simulink model "TEST_IPM_2_0"  (R2019b)
settings: configuration reference "Configuration" (kept outside this file)
PreLoadFcn:
  | RTWConfigurationCB('preloadfcn', bdroot);
values from neighbouring files (symbols this model uses):
  MParamFbase = 200.0    [TEST_IPM_LIB.sldd]
  MParamIbase = 360.0    [TEST_IPM_LIB.sldd]
  MParamLd = 0.002    [TEST_IPM_LIB.sldd]
  MParamLq = 0.002    [TEST_IPM_LIB.sldd]
  MParamRs = 1.15    [TEST_IPM_LIB.sldd]
  PWM_TPBRD_HALF = 5000.0    [TEST_IPM_LIB.sldd]
  Ts_10kHz = 0.0001    [TEST_IPM_LIB.sldd]
  Ts_1kHz = 0.001    [TEST_IPM_LIB.sldd]
undefined symbols (not defined in the file or in its folder): Down, GPTRIP1SEL, GPTRIP2SEL, TZ1, TZ2, Up
libraries: c280xlib x66, c2837xDlib x18, c2802xlib x10, powerlib_meascontrol x9, dsparch4 x4, c2000lib x1, c2806xlib x1, idelinklib_common x1
(part 5 of 6)

== system TEST_IPM_2_0/INT/Read Rotor Position/SpeedCal1 ==
  In1 : Inport
  function : TriggerPort  TriggerType=function-call  VariantControl=Variant
  "First Order Filter " : Subsystem
  MATLAB Function1 : MATLAB Function  TreatAsAtomicUnit=on
  Unit Delay : UnitDelay  SampleTime=-1  HasFrameUpgradeWarning=on
  Out1 : Outport
  wires:
  In1/1 -> Unit Delay/1, MATLAB Function1/1(theta)
  Unit Delay/1 -> MATLAB Function1/2(theta_old)
  MATLAB Function1/1(speed) -> "First Order Filter "/1(input)
  "First Order Filter "/1("output ") -> Out1/1

== system TEST_IPM_2_0/INT/ePWM/If Action Subsystem ==
  Action Port : ActionPort  ActionPortLabel=if(u1 == 1)
  Constant : Constant  Value=0  OutDataTypeStr=single  SampleTime=-1
  Data Store Write : DataStoreWrite  DataStoreName=N_Integral
  Data Store Write1 : DataStoreWrite  DataStoreName=Iq_Integral
  Data Store Write2 : DataStoreWrite  DataStoreName=Id_Integral
  Data Store Write3 : DataStoreWrite  DataStoreName=PLL_Integral
  Data Store Write4 : DataStoreWrite  DataStoreName=Theta_Integral
  wires:
  Constant/1 -> Data Store Write3/1, Data Store Write4/1, Data Store Write1/1, Data Store Write2/1, Data Store Write/1

== system TEST_IPM_2_0/INT/Motor Control/Current_PI/PID_Id  ==
  Ref : Inport
  Fbk : Inport  Port=2
  Data Store Read : DataStoreRead  DataStoreName=Id_Kp
  Data Store Read1 : DataStoreRead  DataStoreName=Id_Integral
  Data Store Read3 : DataStoreRead  DataStoreName=UDCPROTECT
  Data Store Write : DataStoreWrite  DataStoreName=Id_Integral
  MATLAB Function1 : MATLAB Function  TreatAsAtomicUnit=on
  Product : Product  OutDataTypeStr=Inherit: Same as first input
  Subsystem : Subsystem
  Sum1 : Sum  OutDataTypeStr=single
  Sum2 : Sum  Inputs=+-  OutDataTypeStr=Inherit: Inherit via back propagation
  Out : Outport
  wires:
  Data Store Read1/1 -> Subsystem/1(OLD_UI_REG3)
  Fbk/1 -> Sum2/2
  Ref/1 -> Sum2/1
  Product/1 -> Sum1/1
  Data Store Read/1 -> Product/2
  Sum2/1 -> Subsystem/2(up_reg3), Product/1
  Sum1/1 -> Out/1
  Data Store Read3/1 -> MATLAB Function1/1(Udc)
  Subsystem/1(UI_REG1) -> MATLAB Function1/2(Input), Sum1/2
  MATLAB Function1/1(Output) -> Data Store Write/1

== system TEST_IPM_2_0/INT/Motor Control/Current_PI/PID_Iq ==
  Ref : Inport
  Fbk : Inport  Port=2
  Data Store Read : DataStoreRead  DataStoreName=Iq_Kp
  Data Store Read1 : DataStoreRead  DataStoreName=Iq_Integral
  Data Store Read2 : DataStoreRead  DataStoreName=UDCPROTECT
  Data Store Read3 : DataStoreRead  DataStoreName=UDCPROTECT
  Data Store Write : DataStoreWrite  DataStoreName=Iq_Integral
  MATLAB Function : MATLAB Function  TreatAsAtomicUnit=on
  MATLAB Function1 : MATLAB Function  TreatAsAtomicUnit=on
  Product : Product  OutDataTypeStr=Inherit: Same as first input
  Subsystem : Subsystem
  Sum1 : Sum  OutDataTypeStr=single
  Sum2 : Sum  Inputs=+-  OutDataTypeStr=Inherit: Inherit via back propagation
  Out : Outport
  wires:
  MATLAB Function1/1(Output) -> Data Store Write/1
  Subsystem/1(UI_REG1) -> Sum1/2, MATLAB Function1/2(Input)
  Data Store Read3/1 -> MATLAB Function1/1(Udc)
  MATLAB Function/1(Output) -> Out/1
  Data Store Read2/1 -> MATLAB Function/1(Udc)
  Sum1/1 -> MATLAB Function/2(Input)
  Sum2/1 -> Product/1, Subsystem/2(up_reg3)
  Data Store Read/1 -> Product/2
  Product/1 -> Sum1/1
  Ref/1 -> Sum2/1
  Fbk/1 -> Sum2/2
  Data Store Read1/1 -> Subsystem/1(OLD_UI_REG3)

== system TEST_IPM_2_0/INT/Motor Control/Current_PI/RealVoltageCompesation  ==
  Udq : Inport
  Iuvw : Inport  Port=2
  Add : Sum  Inputs=+-
  Add1 : Sum  Inputs=+-
  Add2 : Sum  AccumDataTypeStr=single  OutDataTypeStr=single
  Clark Transformation : Subsystem
  Data Store Read : DataStoreRead  DataStoreName=K
  Data Store Read1 : DataStoreRead  DataStoreName=Udelta
  Data Store Read2 : DataStoreRead  DataStoreName=ControlAng
  Data Store Read3 : DataStoreRead  DataStoreName=N_REF
  Data Store Read4 : DataStoreRead  DataStoreName=DEKF_Udelay
  Data Store Read5 : DataStoreRead  DataStoreName=Alpha_Current
  Data Store Read6 : DataStoreRead  DataStoreName=Beta_Current
  Delay : Delay
  Demux : Demux  Outputs=3
  Demux1 : Demux  Outputs=2
  Gain : Gain  Gain=5/60*2*pi*1e-4
  MATLAB Function : MATLAB Function  TreatAsAtomicUnit=on
  MATLAB Function1 : MATLAB Function  TreatAsAtomicUnit=on
  MATLAB Function2 : MATLAB Function  TreatAsAtomicUnit=on
  Park Transformation : Subsystem
  Park Transformation1 : Subsystem
  Product : Product
  Sqrt : Sqrt  OutputSignalType=real  OutDataTypeStr=single  IntermediateResultsDataTypeStr=single  SaturateOnIntegerOverflow=on
  Square : Math  Operator=square  SignedPower=off  OutputSignalType=real  OutDataTypeStr=single  SaturateOnIntegerOverflow=on
  Square1 : Math  Operator=square  SignedPower=off  OutputSignalType=real  OutDataTypeStr=single  SaturateOnIntegerOverflow=on
  Subsystem : Subsystem
  UdComP : Outport
  UqComP : Outport  Port=2
  UsComP : Outport  Port=3
  wires:
  Udq/1 -> Delay/1
  Demux/1 -> MATLAB Function/1(I)
  Demux/2 -> MATLAB Function1/1(I)
  Demux/3 -> MATLAB Function2/1(I)
  Data Store Read/1 -> MATLAB Function2/2(K), MATLAB Function1/2(K), MATLAB Function/2(K)
  Data Store Read1/1 -> MATLAB Function/3(Udead), MATLAB Function1/3(Udead), MATLAB Function2/3(Udead)
  MATLAB Function/1(Uerror) -> Clark Transformation/1(U)
  MATLAB Function1/1(Uerror) -> Clark Transformation/2(V)
  MATLAB Function2/1(Uerror) -> Clark Transformation/3(W)
  Clark Transformation/2(Beta) -> Park Transformation/2(Beta)
  Delay/1 -> Demux1/1
  Park Transformation/1(D) -> Add/2
  Park Transformation/2(Q) -> Add1/2
  Data Store Read3/1 -> Gain/1
  Demux1/1 -> Park Transformation1/1(Alpha)
  Demux1/2 -> Park Transformation1/2(Beta)
  Sqrt/1 -> UsComP/1
  Square1/1 -> Add2/2
  Add/1 -> Square/1, Subsystem/1(Ud), UdComP/1
  Square/1 -> Add2/1
  Add1/1 -> Subsystem/2(Uq), Square1/1, UqComP/1
  Add2/1 -> Sqrt/1
  Park Transformation1/1(D) -> Add/1
  Park Transformation1/2(Q) -> Add1/1
  Iuvw/1 -> Demux/1
  Data Store Read2/1 -> Subsystem/5(Theta), Park Transformation/3(theta)
  Product/1 -> Park Transformation1/3(theta)
  Gain/1 -> Product/1
  Data Store Read4/1 -> Product/2
  Clark Transformation/1(Alpha) -> Park Transformation/1(Alpha)
  Data Store Read5/1 -> Subsystem/3(Ial)
  Data Store Read6/1 -> Subsystem/4(Ibe)

== system TEST_IPM_2_0/INT/Motor Control/IF/Subsystem1 ==
  TargetValue : Inport
  Step : Inport  Port=2
  MATLAB Function : MATLAB Function  TreatAsAtomicUnit=on
  Unit Delay : UnitDelay  SampleTime=-1  HasFrameUpgradeWarning=on
  RampOutput : Outport
  wires:
  TargetValue/1 -> MATLAB Function/1(Target)
  MATLAB Function/1(Output) -> RampOutput/1, Unit Delay/1
  Step/1 -> MATLAB Function/2(Step)
  Unit Delay/1 -> MATLAB Function/3(LastOutput)

== system TEST_IPM_2_0/INT/Motor Control/IF/Subsystem2 ==
  FRQ : Inport
  MATLAB Function : MATLAB Function  TreatAsAtomicUnit=on
  Unit Delay : UnitDelay  SampleTime=-1  HasFrameUpgradeWarning=on
  Ang : Outport
  wires:
  MATLAB Function/1(Ang) -> Ang/1, Unit Delay/1
  Unit Delay/1 -> MATLAB Function/2(LastAng)
  FRQ/1 -> MATLAB Function/1(FRQ)

== system TEST_IPM_2_0/INT/Motor Control/SVPWM/Inverse Park Transformation ==
  D : Inport
  Q : Inport  Port=2
  theta : Inport  Port=3
  Product{,1..3} (4 alike) : Product  OutDataTypeStr=Inherit: Same as first input
  Sin : Trigonometry  OutputSignalType=real
  Sin1 : Trigonometry  Operator=cos  OutputSignalType=real
  Sum1 : Sum  Inputs=|++  OutDataTypeStr=Inherit: Same as first input
  Sum2 : Sum  Inputs=|+-  OutDataTypeStr=Inherit: Same as first input
  Alpha : Outport
  Beta : Outport  Port=2
  wires:
  Sin1/1 -> Product2/2, Product/2
  Sin/1 -> Product3/2, Product1/2
  Product3/1 -> Sum1/2
  Sum1/1 -> Beta/1
  D/1 -> Product3/1, Product/1
  Product2/1 -> Sum1/1
  Sum2/1 -> Alpha/1
  Product/1 -> Sum2/1
  Product1/1 -> Sum2/2
  Q/1 -> Product2/1, Product1/1
  theta/1 -> Sin/1, Sin1/1

== system TEST_IPM_2_0/INT/Motor Control/SpeedMode/Function-Call Subsystem ==
  function : TriggerPort  TriggerType=function-call  VariantControl=Variant
  Constant : Constant  Value=0  OutDataTypeStr=single  SampleTime=-1
  Constant1 : Constant  Value=0  OutDataTypeStr=single  SampleTime=-1
  Data Store Read1 : DataStoreRead  DataStoreName=N_FBK
  Data Store Read2 : DataStoreRead  DataStoreName=STOP
  Data Store Read3 : DataStoreRead  DataStoreName=N_REF
  Data Store Read5 : DataStoreRead  DataStoreName=FLAG_MTPA
  Data Store Write1 : DataStoreWrite  DataStoreName=Iq_REF
  Demux : Demux  Outputs=2
  If Action Subsystem : Subsystem  TreatAsAtomicUnit=on
  MATLAB Function : MATLAB Function  TreatAsAtomicUnit=on
  Mux : Mux  Inputs=2
  Mux1 : Mux  Inputs=2
  "PID_n " : Subsystem
  Switch : Switch  Criteria=u2 ~= 0
  wires:
  Constant/1 -> Mux1/1
  Constant1/1 -> Mux1/2
  Switch/1 -> Demux/1
  Data Store Read1/1 -> Mux/2
  Demux/2 -> "PID_n "/2(Fbk)
  Demux/1 -> "PID_n "/1(Ref)
  Mux1/1 -> Switch/1
  Data Store Read2/1 -> Switch/2
  Data Store Read3/1 -> Mux/1
  Mux/1 -> Switch/3
  "PID_n "/1(Out) -> Data Store Write1/1
  Data Store Read5/1 -> MATLAB Function/1(FLAG)
  MATLAB Function/1(FcnCal()) -> If Action Subsystem/Trigger

== system TEST_IPM_2_0/INT/Motor Control/TorqueMode/Function-Call Subsystem ==
  function : TriggerPort  TriggerType=function-call  VariantControl=Variant
  Constant : Constant  Value=0  OutDataTypeStr=single  SampleTime=-1
  Constant1 : Constant  Value=0  OutDataTypeStr=single  SampleTime=-1
  Constant2 : Constant  Value=0  OutDataTypeStr=single  SampleTime=-1
  Data Store Write : DataStoreWrite  DataStoreName=N_Integral
  Data Store Write1 : DataStoreWrite  DataStoreName=Iq_Integral
  Data Store Write2 : DataStoreWrite  DataStoreName=Id_Integral
  wires:
  Constant1/1 -> Data Store Write2/1
  Constant2/1 -> Data Store Write1/1
  Constant/1 -> Data Store Write/1

== system TEST_IPM_2_0/INT/Motor Control/VF/Subsystem1 ==
  TargetValue : Inport
  Step : Inport  Port=2
  MATLAB Function : MATLAB Function  TreatAsAtomicUnit=on
  Unit Delay : UnitDelay  SampleTime=-1  HasFrameUpgradeWarning=on
  RampOutput : Outport
  wires:
  TargetValue/1 -> MATLAB Function/1(Target)
  MATLAB Function/1(Output) -> RampOutput/1, Unit Delay/1
  Step/1 -> MATLAB Function/2(Step)
  Unit Delay/1 -> MATLAB Function/3(LastOutput)

== system TEST_IPM_2_0/INT/Motor Control/VF/Subsystem2 ==
  FRQ : Inport
  MATLAB Function : MATLAB Function  TreatAsAtomicUnit=on
  Unit Delay : UnitDelay  SampleTime=-1  HasFrameUpgradeWarning=on
  Ang : Outport
  wires:
  MATLAB Function/1(Ang) -> Ang/1, Unit Delay/1
  Unit Delay/1 -> MATLAB Function/2(LastAng)
  FRQ/1 -> MATLAB Function/1(FRQ)

== system TEST_IPM_2_0/INT/Read Rotor Position/SpeedCal/First Order Filter  ==
  input : Inport
  Add : Sum  Inputs=+-
  Add3 : Sum  AccumDataTypeStr=single
  Constant : Constant  OutDataTypeStr=single  SampleTime=-1
  Data Store Read1 : DataStoreRead  DataStoreName=N_Filter
  Data Store Read2 : DataStoreRead  DataStoreName=N_Filter
  Gain : Gain  Gain=2*pi*Ts_1kHz
  Gain1 : Gain  Gain=2*pi*Ts_1kHz
  Product : Product
  Product1 : Product
  Unit Delay3 : UnitDelay  SampleTime=-1  HasFrameUpgradeWarning=on
  "output " : Outport
  wires:
  input/1 -> Product/1
  Product/1 -> Add3/1
  Product1/1 -> Unit Delay3/1
  Add3/1 -> Product1/1, "output "/1
  Unit Delay3/1 -> Add3/2
  Data Store Read2/1 -> Gain/1
  Gain/1 -> Product/2
  Data Store Read1/1 -> Gain1/1
  Add/1 -> Product1/2
  Gain1/1 -> Add/2
  Constant/1 -> Add/1

== system TEST_IPM_2_0/INT/Read Rotor Position/SpeedCal1/First Order Filter  ==
  input : Inport
  Add : Sum  Inputs=+-
  Add3 : Sum  AccumDataTypeStr=single
  Constant : Constant  OutDataTypeStr=single  SampleTime=-1
  Data Store Read1 : DataStoreRead  DataStoreName=N_Filter
  Data Store Read2 : DataStoreRead  DataStoreName=N_Filter
  Gain : Gain  Gain=2*pi*Ts_1kHz
  Gain1 : Gain  Gain=2*pi*Ts_1kHz
  Product : Product
  Product1 : Product
  Unit Delay3 : UnitDelay  SampleTime=-1  HasFrameUpgradeWarning=on
  "output " : Outport
  wires:
  input/1 -> Product/1
  Product/1 -> Add3/1
  Product1/1 -> Unit Delay3/1
  Add3/1 -> Product1/1, "output "/1
  Unit Delay3/1 -> Add3/2
  Data Store Read2/1 -> Gain/1
  Gain/1 -> Product/2
  Data Store Read1/1 -> Gain1/1
  Add/1 -> Product1/2
  Gain1/1 -> Add/2
  Constant/1 -> Add/1

== system TEST_IPM_2_0/INT/Motor Control/Current_PI/PID_Id /Subsystem ==
  OLD_UI_REG3 : Inport
  up_reg3 : Inport  Port=2
  Data Store Read2 : DataStoreRead  DataStoreName=Id_Ki
  Gain : Gain  Gain=Ts_10kHz
  Product1 : Product  OutDataTypeStr=Inherit: Same as first input
  Sum3 : Sum
  UI_REG1 : Outport
  wires:
  Sum3/1 -> UI_REG1/1
  up_reg3/1 -> Product1/2
  Product1/1 -> Sum3/2
  OLD_UI_REG3/1 -> Sum3/1
  Gain/1 -> Product1/1
  Data Store Read2/1 -> Gain/1

== system TEST_IPM_2_0/INT/Motor Control/Current_PI/PID_Iq/Subsystem ==
  OLD_UI_REG3 : Inport
  up_reg3 : Inport  Port=2
  Data Store Read2 : DataStoreRead  DataStoreName=Iq_Ki
  Gain : Gain  Gain=Ts_10kHz
  Product1 : Product  OutDataTypeStr=Inherit: Same as first input
  Sum3 : Sum
  UI_REG1 : Outport
  wires:
  Data Store Read2/1 -> Gain/1
  Gain/1 -> Product1/1
  OLD_UI_REG3/1 -> Sum3/1
  Product1/1 -> Sum3/2
  up_reg3/1 -> Product1/2
  Sum3/1 -> UI_REG1/1

== system TEST_IPM_2_0/INT/Motor Control/Current_PI/RealVoltageCompesation /Clark Transformation ==
  U : Inport
  V : Inport  Port=2
  W : Inport  Port=3
  Add : Sum  Inputs=+--
  Add1 : Sum  Inputs=+-
  Gain : Gain  Gain=0.5
  Gain1 : Gain  Gain=0.5
  Gain2 : Gain  Gain=2/3
  Gain3 : Gain  Gain=2/3*0.86602540
  Alpha : Outport
  Beta : Outport  Port=2
  wires:
  V/1 -> Add1/1, Gain/1
  Gain/1 -> Add/2
  W/1 -> Add1/2, Gain1/1
  Gain1/1 -> Add/3
  U/1 -> Add/1
  Add/1 -> Gain2/1
  Gain2/1 -> Alpha/1
  Add1/1 -> Gain3/1
  Gain3/1 -> Beta/1

== system TEST_IPM_2_0/INT/Motor Control/Current_PI/RealVoltageCompesation /Park Transformation ==
  Alpha : Inport
  Beta : Inport  Port=2
  theta : Inport  Port=3
  Add : Sum
  Add1 : Sum  Inputs=+-
  Product{,1..3} (4 alike) : Product
  Sin : Trigonometry  OutputSignalType=real
  Sin1 : Trigonometry  Operator=cos  OutputSignalType=real
  D : Outport
  Q : Outport  Port=2
  wires:
  Product/1 -> Add/1
  Sin/1 -> Product3/2, Product1/2
  Product1/1 -> Add/2
  Add1/1 -> Q/1
  Sin1/1 -> Product2/2, Product/2
  Product2/1 -> Add1/1
  Alpha/1 -> Product3/1, Product/1
  Beta/1 -> Product2/1, Product1/1
  Product3/1 -> Add1/2
  Add/1 -> D/1
  theta/1 -> Sin/1, Sin1/1

== system TEST_IPM_2_0/INT/Motor Control/Current_PI/RealVoltageCompesation /Park Transformation1 ==
  Alpha : Inport
  Beta : Inport  Port=2
  theta : Inport  Port=3
  Add : Sum
  Add1 : Sum  Inputs=+-
  Product{,1..3} (4 alike) : Product
  Sin : Trigonometry  OutputSignalType=real
  Sin1 : Trigonometry  Operator=cos  OutputSignalType=real
  D : Outport
  Q : Outport  Port=2
  wires:
  theta/1 -> Sin1/1, Sin/1
  Add/1 -> D/1
  Product3/1 -> Add1/2
  Beta/1 -> Product1/1, Product2/1
  Alpha/1 -> Product/1, Product3/1
  Product2/1 -> Add1/1
  Sin1/1 -> Product/2, Product2/2
  Add1/1 -> Q/1
  Product1/1 -> Add/2
  Sin/1 -> Product1/2, Product3/2
  Product/1 -> Add/1

== system TEST_IPM_2_0/INT/Motor Control/Current_PI/RealVoltageCompesation /Subsystem ==
  Ud : Inport
  Uq : Inport  Port=2
  Ial : Inport  Port=3
  Ibe : Inport  Port=4
  Theta : Inport  Port=5
  Data Store Read : DataStoreRead  DataStoreName=SMO_EalEstOut
  Data Store Read1 : DataStoreRead  DataStoreName=SMO_EbeEstOut
  Data Store Read2 : DataStoreRead  DataStoreName=ResloverAng
  Data Store Write : DataStoreWrite  DataStoreName=SMO_Ual
  Data Store Write1 : DataStoreWrite  DataStoreName=SMO_Ube
  Data Store Write11 : DataStoreWrite  DataStoreName=SMO_Theta
  Data Store Write2 : DataStoreWrite  DataStoreName=SMO_Ial
  Data Store Write3 : DataStoreWrite  DataStoreName=SMO_Ibe
  Data Store Write4 : DataStoreWrite  DataStoreName=SMO_Error
  Data Store Write5 : DataStoreWrite  DataStoreName=SMO_EamEst
  Inverse Park Transformation : Subsystem
  MATLAB Function3 : MATLAB Function  TreatAsAtomicUnit=on
      settings: RTWSystemCode=Inline
  wires:
  Inverse Park Transformation/2(Beta) -> Data Store Write1/1
  MATLAB Function3/1(Theta) -> Data Store Write11/1
  Uq/1 -> Inverse Park Transformation/2(Q)
  Ibe/1 -> Data Store Write3/1
  Inverse Park Transformation/1(Alpha) -> Data Store Write/1
  Ial/1 -> Data Store Write2/1
  Theta/1 -> Inverse Park Transformation/3(theta)
  Ud/1 -> Inverse Park Transformation/1(D)
  Data Store Read2/1 -> MATLAB Function3/3(ControlAng)
  MATLAB Function3/2(Error) -> Data Store Write4/1
  MATLAB Function3/3(Eam) -> Data Store Write5/1
  Data Store Read/1 -> MATLAB Function3/1(Eal)
  Data Store Read1/1 -> MATLAB Function3/2(Ebe)

== system TEST_IPM_2_0/INT/Motor Control/SpeedMode/Function-Call Subsystem/If Action Subsystem ==
  function : TriggerPort  TriggerType=function-call  VariantControl=Variant
  Abs : Abs
  Data Store Read : DataStoreRead  DataStoreName=MTPA_Gamma
  Data Store Read3 : DataStoreRead  DataStoreName=Iq_REF
  Data Store Write1 : DataStoreWrite  DataStoreName=Iq_REF
  Data Store Write2 : DataStoreWrite  DataStoreName=Id_REF
  Gain1 : Gain  Gain=-1  OutDataTypeStr=single
  Product : Product  OutDataTypeStr=single
  Product1 : Product  OutDataTypeStr=single
  Saturation : Saturate  UpperLimit=pi/2  LowerLimit=0
  cos : Trigonometry  Operator=cos  OutputSignalType=real
  sin : Trigonometry  OutputSignalType=real
  wires:
  sin/1 -> Product1/1
  Abs/1 -> Gain1/1
  cos/1 -> Product/2
  Saturation/1 -> sin/1, cos/1
  Product/1 -> Data Store Write1/1
  Gain1/1 -> Product1/2
  Data Store Read3/1 -> Abs/1, Product/1
  Product1/1 -> Data Store Write2/1
  Data Store Read/1 -> Saturation/1

== system TEST_IPM_2_0/INT/Motor Control/SpeedMode/Function-Call Subsystem/PID_n  ==
  Ref : Inport
  Fbk : Inport  Port=2
  Constant : Constant  Value=MParamIbase  OutDataTypeStr=single  SampleTime=-1
  Data Store Read : DataStoreRead  DataStoreName=N_Kp
  Data Store Read1 : DataStoreRead  DataStoreName=N_Integral
  Data Store Write : DataStoreWrite  DataStoreName=N_Integral
  MATLAB Function : MATLAB Function  TreatAsAtomicUnit=on
  Product : Product  OutDataTypeStr=Inherit: Same as first input
  Subsystem : Subsystem
  Sum1 : Sum  OutDataTypeStr=single
  Sum2 : Sum  Inputs=+-  OutDataTypeStr=Inherit: Inherit via back propagation
  Out : Outport
  wires:
  Data Store Read1/1 -> Subsystem/1(OLD_UI_REG3)
  Fbk/1 -> Sum2/2
  Ref/1 -> Sum2/1
  Product/1 -> Sum1/1
  Data Store Read/1 -> Product/2
  Subsystem/1(UI_REG1) -> Data Store Write/1, Sum1/2
  Sum2/1 -> Subsystem/2(up_reg3), Product/1
  MATLAB Function/1(Output) -> Out/1
  Sum1/1 -> MATLAB Function/2(Input)
  Constant/1 -> MATLAB Function/1(Limit)

== system TEST_IPM_2_0/INT/Motor Control/Current_PI/RealVoltageCompesation /Subsystem/Inverse Park Transformation ==
  D : Inport
  Q : Inport  Port=2
  theta : Inport  Port=3
  Product{,1..3} (4 alike) : Product  OutDataTypeStr=Inherit: Same as first input
  Sin : Trigonometry  OutputSignalType=real
  Sin1 : Trigonometry  Operator=cos  OutputSignalType=real
  Sum1 : Sum  Inputs=|++  OutDataTypeStr=Inherit: Same as first input
  Sum2 : Sum  Inputs=|+-  OutDataTypeStr=Inherit: Same as first input
  Alpha : Outport
  Beta : Outport  Port=2
  wires:
  Sin1/1 -> Product2/2, Product/2
  Sin/1 -> Product3/2, Product1/2
  Product3/1 -> Sum1/2
  Sum1/1 -> Beta/1
  D/1 -> Product3/1, Product/1
  Product2/1 -> Sum1/1
  Sum2/1 -> Alpha/1
  Product/1 -> Sum2/1
  Product1/1 -> Sum2/2
  Q/1 -> Product2/1, Product1/1
  theta/1 -> Sin/1, Sin1/1

== system TEST_IPM_2_0/INT/Motor Control/SpeedMode/Function-Call Subsystem/PID_n /Subsystem ==
  OLD_UI_REG3 : Inport
  up_reg3 : Inport  Port=2
  Data Store Read2 : DataStoreRead  DataStoreName=N_Ki
  Gain : Gain  Gain=Ts_1kHz
  Product1 : Product  OutDataTypeStr=Inherit: Same as first input
  Sum3 : Sum  OutDataTypeStr=single
  UI_REG1 : Outport
  wires:
  Sum3/1 -> UI_REG1/1
  up_reg3/1 -> Product1/2
  Product1/1 -> Sum3/2
  OLD_UI_REG3/1 -> Sum3/1
  Gain/1 -> Product1/1
  Data Store Read2/1 -> Gain/1

== stateflow chart TEST_IPM_2_0/INT/AD2S1210 Init/AD2S1210 ==
  settings: updateMethod=DISCRETE  initializeOutput=1
  state Empty
    entry:
    Wait_Count = 0;
  state RESET_STEP1
    entry:
    Wait_Count  = Wait_Count + 1;
    ResloverRESET = 0;
    EV_RESET();
  state RESET_STEP2
    entry:
    ResloverRESET = 1;
    EV_RESET();
  state INIT_ConfigMode
    entry:
    ResloverA0=1;
    ResloverA1=1;
    ConfigMode();
  state WRITE_FRQ_STEP1
    entry:
    ResloverWR=1;
    WRITE_SPI_STEP1();
  state WRITE_FRQ_STEP4
    entry:
    ResloverWR=1;
    WRITE_SPI_STEP1();
  state READ_FAULT_STEP1
    entry:
    ResloverWR=1;
    WRITE_SPI_STEP1();
  state READ_FAULT_STEP4
    entry:
    ResloverWR=1;
    WRITE_SPI_STEP1();
  state READ_FAULT_STEP5
    entry:
    ResloverWR=1;
    WRITE_SPI_STEP1();
  state WRITE_FRQ_STEP2
    entry:
    ResloverWR=0;
    SPIC_Tx=uint16(hex2dec('9191'));
    WRITE_SPI_STEP2();
  state WRITE_FRQ_STEP5
    entry:
    ResloverWR=0;
    SPIC_Tx=ResloverFRQ*256+ResloverFRQ;
    WRITE_SPI_STEP2();
  state READ_FAULT_STEP2
    entry:
    ResloverWR=0;
    SPIC_Tx=uint16(hex2dec('FFFF'));
    WRITE_SPI_STEP2();
  state READ_FAULT_STEP3
    entry:
    ResloverWR=0;
    SPIC_Tx=uint16(hex2dec('FFFF'));
    WRITE_SPI_STEP2();
  state READ_FAULT_STEP6
    entry:
    ResloverWR=0;
    SPIC_Tx=uint16(hex2dec('FFFF'));
    WRITE_SPI_STEP2();
  state WRITE_RES_STEP1
    entry:
    ResloverWR=1;
    WRITE_SPI_STEP1();
  state WRITE_RES_STEP3
    entry:
    ResloverWR=1;
    WRITE_SPI_STEP1();
  state WRITE_RES_STEP2
    entry:
    ResloverWR=0;
    SPIC_Tx=uint16(hex2dec('9292'));
    WRITE_SPI_STEP2();
  state WRITE_RES_STEP4
    entry:
    ResloverWR=0;
    SPIC_Tx=ResloverRES*256+ResloverRES;
    WRITE_SPI_STEP2();
  state INIT_FINISH
    entry:
    ResloverWR=0;
    ResloverA0=0;
    ResloverA1=0;
    InitMode=2;
    INIT_FINISH();
  (default) -> Empty
  Empty -> RESET_STEP1 : [InitMode==1]
  RESET_STEP1 -> RESET_STEP1 [order 2]
  RESET_STEP1 -> RESET_STEP2 [order 1] : [Wait_Count > 1000]
  INIT_FINISH -> RESET_STEP2
  RESET_STEP2 -> INIT_ConfigMode : [InitMode==1]
  INIT_ConfigMode -> WRITE_FRQ_STEP1
  WRITE_FRQ_STEP2 -> WRITE_FRQ_STEP4
  READ_FAULT_STEP2 -> READ_FAULT_STEP4
  WRITE_RES_STEP4 -> READ_FAULT_STEP1
  READ_FAULT_STEP3 -> READ_FAULT_STEP5
  WRITE_FRQ_STEP1 -> WRITE_FRQ_STEP2
  WRITE_FRQ_STEP4 -> WRITE_FRQ_STEP5
  READ_FAULT_STEP1 -> READ_FAULT_STEP2
  READ_FAULT_STEP4 -> READ_FAULT_STEP3
  READ_FAULT_STEP5 -> READ_FAULT_STEP6
  WRITE_FRQ_STEP5 -> WRITE_RES_STEP1
  READ_FAULT_STEP6 -> INIT_FINISH
  WRITE_RES_STEP2 -> WRITE_RES_STEP3
  WRITE_RES_STEP1 -> WRITE_RES_STEP2
  WRITE_RES_STEP3 -> WRITE_RES_STEP4
  data: ResloverWR data_store_memory; ResloverRESET data_store_memory; SPIC_Tx data_store_memory; ResloverA0 data_store_memory; ResloverA1 data_store_memory; ResloverFRQ data_store_memory; InitMode data_store_memory; ResloverRES data_store_memory; Wait_Count local
  events: EV_RESET output FUNCTION_CALL_EVENT; ConfigMode output FUNCTION_CALL_EVENT; WRITE_SPI_STEP1 output FUNCTION_CALL_EVENT; WRITE_SPI_STEP2 output FUNCTION_CALL_EVENT; INIT_FINISH output FUNCTION_CALL_EVENT

== matlab function TEST_IPM_2_0/INT/Current Bias Init/MATLAB Function ==
  data: InitMode output
function InitMode = TICK_ADD
persistent Tick
if isempty(Tick)
    Tick = uint16(0);
end
Tick = Tick + uint16(1);
if(Tick <= 50000)
    InitMode = uint16(2);
else
    InitMode = uint16(0);
    Tick = uint16(0);
end
end

== stateflow chart TEST_IPM_2_0/INT/Chart ==
  settings: updateMethod=DISCRETE  initializeOutput=1  enableNonTerminalStates=1
  state Empty
  state Init
    entry:
    ADCINT_IN();
  state ADC_Sample
    entry:
    ADCSample();
    ResloverSAMPLE=0;
  state AD2S1210
    entry:
    SPIC_Tx = 0;
    ResloverSAMPLE=1;
    AD2S1210();
  state System_InitADBias
    entry:
    STOP=1;
    INIT_ADBias();
  state System_InitAD2S1210
    entry:
    STOP=1;
    INIT_AD2S1210();
  state MOTORCONTROL
    entry:
    MOTORCONTROL();
  state Extra_Observer
    entry:
    Extra_Observer();
  state ePWM
    entry:
    ePWM();
  state BufferStore
    entry:
    Buffer();
  state DA_5742
    entry:
    DA_5742();
  state end
    entry:
    ADCINT_OUT();
    ChartFlag= 1;
  (default) -> Empty
  end -> Empty
  Empty -> Init : [ChartFlag==0]
  Init -> ADC_Sample
  ADC_Sample -> System_InitAD2S1210 [order 2] : [InitMode==1]
  ADC_Sample -> System_InitADBias [order 3] : [InitMode==2]
  ADC_Sample -> AD2S1210 [order 1] : [InitMode==0]
  AD2S1210 -> MOTORCONTROL
  System_InitAD2S1210 -> ePWM
  System_InitADBias -> ePWM
  MOTORCONTROL -> Extra_Observer [order 2]
  MOTORCONTROL -> ePWM [order 1] : [DEKF_FLAG == 0]
  Extra_Observer -> ePWM
  ePWM -> BufferStore
  BufferStore -> DA_5742
  DA_5742 -> end
  data: InitMode data_store_memory; ChartFlag data_store_memory; ResloverSAMPLE data_store_memory; SPIC_Tx data_store_memory; STOP data_store_memory; DEKF_FLAG data_store_memory
  events: ADCINT_IN output FUNCTION_CALL_EVENT; ADCSample output FUNCTION_CALL_EVENT; INIT_AD2S1210 output FUNCTION_CALL_EVENT; INIT_ADBias output FUNCTION_CALL_EVENT; AD2S1210 output FUNCTION_CALL_EVENT; MOTORCONTROL output FUNCTION_CALL_EVENT; Extra_Observer output FUNCTION_CALL_EVENT; ePWM output FUNCTION_CALL_EVENT; Buffer output FUNCTION_CALL_EVENT; DA_5742 output FUNCTION_CALL_EVENT; ADCINT_OUT output FUNCTION_CALL_EVENT

== matlab function TEST_IPM_2_0/INT/Read Rotor Position/MATLAB Function ==
  events: FunCall output FUNCTION_CALL_EVENT
function SpeedDivder
persistent Tick
if isempty(Tick)
    Tick = uint16(0);
end
Tick = Tick + uint16(1);
if(Tick == 10)
    Tick = uint16(0);
    FunCall;
end

== matlab function TEST_IPM_2_0/INT/Current Sampling/MATLAB Function ==
  data: U input; V input; W input; PROTECT data_store_memory; STOP data_store_memory
function Current_Protect(U,V,W)
global PROTECT STOP
if (U>25||U<-25||V>25||V<-25||W>25||W<-25)
    STOP = uint16(1);
    PROTECT = uint16(bitor(PROTECT,1)); 
end

if(PROTECT ~= uint16(0))
    STOP = uint16(1);
end

== matlab function TEST_IPM_2_0/INT/Motor Control/SpeedMode/MATLAB Function ==
  events: Speed_PI output FUNCTION_CALL_EVENT
function Count()
persistent count; 
if isempty(count)
    count = uint16(0);
end

count = count + uint16(1);
if(count == 10)
    count = uint16(0);
    Speed_PI();
end

end

== matlab function TEST_IPM_2_0/Temperature&DCBUS/MATLAB Function ==
  data: input input; Output output
function Output = Udc(input)
Output = single((single(input)-single(8))*single(0.147220477));
end

== matlab function TEST_IPM_2_0/INT/Read Rotor Position/RAW_DATA2Angle  ==
  data: Raw_Data input; Angle_out output; Mech_Theta_out output; Mid_Position input
function [Angle_out,Mech_Theta_out] = Raw_Data2Angle(Raw_Data,Mid_Position)
    Angle = single(Raw_Data) - single(Mid_Position);
    if(Angle < 0)
        Angle = Angle + single(65535);
    end
    Mech_Theta = single(Angle)*single(1)*(single(1.5259e-5));
    Angle = single(Angle)*single(1)*(single(1.5259e-5));
    Angle = mod(Angle,single(1));
    Mech_Theta = mod(Mech_Theta,single(1));
    Angle_out = Angle;
    Mech_Theta_out = Mech_Theta;
end

== matlab function TEST_IPM_2_0/Temperature&DCBUS/MATLAB Function1 ==
  data: input input; Output output
function Output = Temp(input)
temp_voltage=single(input)*single(0.00073242);
Output = single(126.3) - single(198.8)*temp_voltage + single(133.3)*temp_voltage*temp_voltage-single(33.83)*temp_voltage*temp_voltage*temp_voltage;
end

== matlab function TEST_IPM_2_0/Temperature&DCBUS/MATLAB Function2 ==
  data: input input; Output output
function Output = Temp(input)
temp_voltage=single(input)*single(0.00073242);
Output = single(126.3) - single(198.8)*temp_voltage + single(133.3)*temp_voltage*temp_voltage-single(33.83)*temp_voltage*temp_voltage*temp_voltage;
end

== matlab function TEST_IPM_2_0/Temperature&DCBUS/MATLAB Function3 ==
  data: Temp_Max input; UDC input; N_REF input; N_FBK input; PROTECT data_store_memory; STOP data_store_memory; UDCPROTECT data_store_memory; ControlMode input
function PROTECT(Temp_Max,UDC,N_REF,N_FBK,ControlMode)
global PROTECT UDCPROTECT STOP
    if(Temp_Max >= 85)
        PROTECT = uint16(bitor(PROTECT,uint16(4)));
        STOP = uint16(1);
    end
    if(UDC >= UDCPROTECT + 40 ||UDC <= UDCPROTECT - 40)
        PROTECT = uint16(bitor(PROTECT,uint16(2)));
        STOP = uint16(1);
    end    

    if((N_FBK >= N_REF + single(300)|| N_FBK<= N_REF - single(300))&&ControlMode==uint16(4))
         PROTECT = uint16(bitor(PROTECT,uint16(8)));
         STOP = uint16(1);
    end
end

== matlab function TEST_IPM_2_0/Temperature&DCBUS/MATLAB Function4 ==
  data: input input; Output output
function Output = Temp(input)
temp_voltage=single(input)*single(0.00073242);
Output = single(126.3) - single(198.8)*temp_voltage + single(133.3)*temp_voltage*temp_voltage-single(33.83)*temp_voltage*temp_voltage*temp_voltage;
end

== matlab function TEST_IPM_2_0/INT/Motor Control/IF/Subsystem1/MATLAB Function ==
  data: Target input single; Output output; Step input single; LastOutput input single
function Output = RAMPCONTROL(Target,Step,LastOutput)
if(LastOutput <= Target)
    Temp = LastOutput + Step;
else
    Temp = LastOutput - Step;
end
if (abs(Temp - Target) <= Step * 2)
    Temp = Target;
end
    Output = Temp;
end

== matlab function TEST_IPM_2_0/INT/Motor Control/SpeedMode/Function-Call Subsystem/PID_n /MATLAB Function ==
  data: Limit input; Input input; Output output
function Output = Saturation(Limit,Input)
if(Input >= Limit)
    Output = Limit;
elseif(Input <= -Limit)
    Output = -Limit;
else
    Output = Input;
end

== matlab function TEST_IPM_2_0/INT/Motor Control/VF/Subsystem1/MATLAB Function ==
  data: Target input single; Output output; Step input single; LastOutput input single
function Output = RAMPCONTROL(Target,Step,LastOutput)
if(LastOutput <= Target)
    Temp = LastOutput + Step;
else
    Temp = LastOutput - Step;
end
if (abs(Temp - Target) <= Step * 2)
    Temp = Target;
end
    Output = Temp;
end

== matlab function TEST_IPM_2_0/INT/Motor Control/TorqueMode/MATLAB Function3 ==
  data: ThetaEst input; ThetaOut output; FLAG input; ThetaReal input; nREF input
function ThetaOut = ThetaSwitch(ThetaEst,FLAG,ThetaReal,nREF)
if(FLAG == uint16(1))
    ThetaOut = ThetaEst;
elseif(FLAG == uint16(2))
    if(nREF <= single(3.6))
        ThetaOut = ThetaEst;
    else
        ThetaOut = ThetaReal;
    end
else
    ThetaOut = ThetaReal;
end

== matlab function TEST_IPM_2_0/INT/Motor Control/VF/Subsystem2/MATLAB Function ==
  data: FRQ input single; Ang output; LastAng input single
function Ang = AngOutput(FRQ,LastAng)
    Temp = LastAng + FRQ*single(1e-4 * 2* pi);
    if(Temp > single(2*pi))
        Temp = Temp - single(2*pi);
    end
    Ang = Temp;
end

== matlab function TEST_IPM_2_0/INT/Motor Control/IF/Subsystem2/MATLAB Function ==
  data: FRQ input single; Ang output; LastAng input single
function Ang = AngOutput(FRQ,LastAng)
    Temp = LastAng + FRQ*single(1e-4 * 2* pi);
    if(Temp > single(2*pi))
        Temp = Temp - single(2*pi);
    end
    Ang = Temp;
end

== matlab function TEST_IPM_2_0/INT/Motor Control/Current_PI/PID_Id /MATLAB Function1 ==
  data: Udc input; Output output; Input input
function Output = Saturation(Udc,Input)
if(Input >= Udc/sqrt(3))
    Output = Udc/sqrt(3);
elseif(Input <= -Udc/sqrt(3))
    Output = -Udc/sqrt(3);
else
    Output = Input;
end

== matlab function TEST_IPM_2_0/INT/Motor Control/Current_PI/MATLAB Function1 ==
  data: Ud input; Uq input; Ud_out output; Us_out output; Uq_out output; ControlMode data_store_memory; VF_Ud data_store_memory; VF_Uq data_store_memory; UDCPROTECT input; STOP data_store_memory
function [Ud_out,Us_out,Uq_out] = Over_Modulation(Ud,Uq,UDCPROTECT)
global ControlMode VF_Ud VF_Uq;
global STOP;
Us = sqrt(Ud*Ud+Uq*Uq);
Us_out = Us;
if(Us>UDCPROTECT/sqrt(3))
    Ud_out_temp = Ud/Us*Ud;
    Uq_out_temp = Uq/Us*Uq;
else
    Ud_out_temp = Ud;
    Uq_out_temp = Uq;
end
    
if(ControlMode == 1)
    Ud_out = VF_Ud;
    Uq_out = VF_Uq;
else
    Ud_out = Ud_out_temp;
    Uq_out = Uq_out_temp;
end

if(STOP ~= 0)
    Ud_out = single(0);
    Uq_out = single(0); 
    Us_out = single(0); 
end    
end

== matlab function TEST_IPM_2_0/INT/Motor Control/Current_PI/MATLAB Function ==
  data: Udc input; Output output; Input input
function Output = Saturation(Udc,Input)
if(Input >= Udc/sqrt(3))
    Output = Udc/sqrt(3);
elseif(Input <= -Udc/sqrt(3))
    Output = -Udc/sqrt(3);
else
    Output = Input;
end

== matlab function TEST_IPM_2_0/INT/Motor Control/Current_PI/PID_Iq/MATLAB Function ==
  data: Udc input; Output output; Input input
function Output = Saturation(Udc,Input)
if(Input >= Udc/sqrt(3))
    Output = Udc/sqrt(3);
elseif(Input <= -Udc/sqrt(3))
    Output = -Udc/sqrt(3);
else
    Output = Input;
end

== matlab function TEST_IPM_2_0/INT/Motor Control/Current_PI/PID_Iq/MATLAB Function1 ==
  data: Udc input; Output output; Input input
function Output = Saturation(Udc,Input)
if(Input >= Udc/sqrt(3))
    Output = Udc/sqrt(3);
elseif(Input <= -Udc/sqrt(3))
    Output = -Udc/sqrt(3);
else
    Output = Input;
end

== matlab function TEST_IPM_2_0/INT/Motor Control/SVPWM/MATLAB Function ==
  data: alpha input; ta output; beta input; tb output; tc output
function [ta,tb,tc] = SVPWM(alpha,beta)

temp1=beta;
temp2=0.5*beta+0.86603*alpha;
temp3=temp2-temp1;

VecSector=3;
if(temp2>0)
    VecSector=VecSector-1;
end
if(temp3>0)
    VecSector=VecSector-1;
end
if(temp1<0)
    VecSector=7-VecSector;
end

switch VecSector
    case 1
        ta=temp2;
        tb=temp1-temp3;
        tc=-temp2;
    case 2
        ta=temp3+temp2;
        tb=temp1;
        tc=-temp1;
    case 3
        ta=temp3;
        tb=-temp3;
        tc=-(temp1+temp2);
    case 4
        ta=temp2;
        tb=temp1-temp3;
        tc=-temp2;
    case 5
        ta=temp3+temp2;
        tb=temp1;
        tc=-temp1;
    case 6
        ta=temp3;
        tb=-temp3;
        tc=-(temp1+temp2);
    otherwise
        ta=single(0.5);
        tb=single(0.5);
        tc=single(0.5);
end

== matlab function TEST_IPM_2_0/SpeedREF/Subsystem1/MATLAB Function ==
  data: Target input single; Output output; Step input single; LastOutput input single; STOP data_store_memory
function Output = RAMPCONTROL(Target,Step,LastOutput)
global STOP
if(LastOutput <= Target)
    Temp = LastOutput + Step;
else
    Temp = LastOutput - Step;
end
if (abs(Temp - Target) <= Step * 2)
    Temp = Target;
end
if(STOP ~= uint16(0))
    Temp = single(0);
end
    Output = Temp;
    
end

== matlab function TEST_IPM_2_0/INT/Motor Control/Current_PI/RealVoltageCompesation /MATLAB Function ==
  data: I input; Uerror output; K input; Udead input
function Uerror = VSIComp(I,K,Udead)
Uerror = single(2) * Udead * (single(1)/(single(1) + exp(-K*I))-single(0.5));
% Uerror = Udead * atan( I * K ) /(single(pi) * single(0.5));
end

== matlab function TEST_IPM_2_0/INT/Motor Control/Current_PI/RealVoltageCompesation /MATLAB Function1 ==
  data: I input; Uerror output; K input; Udead input
function Uerror = VSIComp(I,K,Udead)
Uerror = single(2) * Udead * (single(1)/(single(1) + exp(-K*I))-single(0.5));
% Uerror = Udead * atan( I * K ) /(single(pi) * single(0.5));
end

== matlab function TEST_IPM_2_0/INT/Motor Control/Current_PI/RealVoltageCompesation /MATLAB Function2 ==
  data: I input; Uerror output; K input; Udead input
function Uerror = VSIComp(I,K,Udead)
Uerror = single(2) * Udead * (single(1)/(single(1) + exp(-K*I))-single(0.5));
% Uerror = Udead * atan( I * K ) /(single(pi) * single(0.5));
end

== matlab function TEST_IPM_2_0/INT/Motor Control/Current_PI/MATLAB Function2 ==
  data: Udc input; Output output; Input input
function Output = Saturation(Udc,Input)
if(Input >= Udc/sqrt(3))
    Output = Udc/sqrt(3);
elseif(Input <= -Udc/sqrt(3))
    Output = -Udc/sqrt(3);
else
    Output = Input;
end

== matlab function TEST_IPM_2_0/BufferOut/MATLAB Function ==
  data: ArrayId_REF data_store_memory; ArrayId_FBK data_store_memory; ArrayIq_REF data_store_memory; ArrayIq_FBK data_store_memory; ArrayUdComP data_store_memory; ArrayUqComP data_store_memory; ArrayTheta data_store_memory; BufferOutId_REF data_store_memory; BufferOutId_FBK data_store_memory; BufferOutUdComP data_store_memory; BufferOutIq_REF data_store_memory; BufferOutIq_FBK data_store_memory; BufferOutUqComP data_store_memory; BufferOutTheta data_store_memory; BufferFlag data_store_memory
function BufferOut
global ArrayId_REF ArrayId_FBK ArrayUdComP 
global ArrayIq_REF ArrayIq_FBK ArrayUqComP
global ArrayTheta
global BufferFlag    
global BufferOutId_REF BufferOutId_FBK BufferOutUdComP
global BufferOutIq_REF BufferOutIq_FBK BufferOutUqComP
global BufferOutTheta
persistent count_out switch_count;

if isempty(count_out)
    count_out =uint16(1);
end
if isempty(switch_count)
    switch_count =uint16(1);
end

if(BufferFlag == 0)
    BufferOutId_REF = single(0);
    BufferOutId_FBK = single(0);
    BufferOutUdComP = single(0);
    BufferOutIq_REF = single(0);
    BufferOutIq_FBK = single(0);
    BufferOutUqComP = single(0);
    BufferOutTheta  = single(0);
else
    if(count_out <= 500)
        switch switch_count
            case 1
                BufferOutId_REF = ArrayId_REF(count_out);
                switch_count = uint16(2);
            case 2
                BufferOutId_FBK = ArrayId_FBK(count_out);
                switch_count = uint16(3);
            case 3
                BufferOutUdComP = ArrayUdComP(count_out);
                switch_count = uint16(4);
            case 4
                BufferOutIq_REF = ArrayIq_REF(count_out);
                switch_count = uint16(5);
            case 5
                BufferOutIq_FBK = ArrayIq_FBK(count_out);
                switch_count = uint16(6);
            case 6
                BufferOutUqComP = ArrayUqComP(count_out);
                switch_count = uint16(7);
            case 7
                BufferOutTheta  =  ArrayTheta(count_out);
                switch_count = uint16(1);
                count_out = count_out + uint16(1);
        end
    else
        BufferOutId_REF = single(0);
        BufferOutId_FBK = single(0);
        BufferOutUdComP = single(0);
        BufferOutIq_REF = single(0);
        BufferOutIq_FBK = single(0);
        BufferOutUqComP = single(0);
        BufferOutTheta  = single(0);   
        count_out = uint16(1);
        BufferFlag = uint16(0);
    end
end    
    
end

== matlab function TEST_IPM_2_0/INT/Data Buffer/Subsystem/MATLAB Function ==
  data: IdREF input; IdFBK input; UdComP input; IqREF input; IqFBK input; UqComP input; Theta input; ArrayId_REF data_store_memory; ArrayId_FBK data_store_memory; ArrayIq_REF data_store_memory; ArrayIq_FBK data_store_memory; ArrayUdComP data_store_memory; ArrayUqComP data_store_memory; ArrayTheta data_store_memory; BufferFlag data_store_memory
function Buffer_In(IdREF,IdFBK,UdComP,IqREF,IqFBK,UqComP,Theta)
global ArrayId_REF ArrayId_FBK ArrayUdComP 
global ArrayIq_REF ArrayIq_FBK ArrayUqComP
global ArrayTheta
global BufferFlag
persistent count
if isempty(count)
	count = uint16(1);
end

if(BufferFlag == 1)
    count = uint16(1);
else
    if(count <= uint16(500))
        ArrayId_REF(count) = single(IdREF);
        ArrayId_FBK(count) = single(IdFBK);
        ArrayUdComP(count) = single(UdComP);
        ArrayIq_REF(count) = single(IqREF);
        ArrayIq_FBK(count) = single(IqFBK);
        ArrayUqComP(count) = single(UqComP);
        ArrayTheta (count) = single(Theta);
        count = count + uint16(1);
    else
        count = uint16(1);
        BufferFlag = uint16(1);
    end
end
end

== stateflow chart TEST_IPM_2_0/INT/MAX5742/MAX5742 ==
  settings: updateMethod=DISCRETE  initializeOutput=1  enableNonTerminalStates=1
  state DAC_A
    entry:
    count_5742 = uint16(0);
    DAC_A_OUT();
  state Wait
    entry:
    count_5742 = count_5742 + uint16(1);
  state DAC_B
    entry:
    count_5742 = uint16(0);
    DAC_B_OUT();
  state empty
  state Wait1
    entry:
    count_5742 = count_5742 + uint16(1);
  state DAC_C
    entry:
    count_5742 = uint16(0);
    DAC_C_OUT();
  state Wait3
    entry:
    count_5742 = count_5742 + uint16(1);
  state DAC_D
    entry:
    FLAG_5742 = uint16(1);
    count_5742 = uint16(0);
    DAC_D_OUT();
  (default) -> DAC_A
  empty -> DAC_A : [FLAG_5742 == 0]
  DAC_A -> (junction 5)
  (junction 5) -> Wait [order 2]
  Wait -> (junction 5)
  (junction 5) -> DAC_B [order 1] : [count_5742 > 20]
  DAC_B -> (junction 15)
  DAC_D -> empty
  (junction 15) -> Wait1 [order 2]
  Wait1 -> (junction 15)
  (junction 15) -> DAC_C [order 1] : [count_5742 > 20]
  DAC_C -> (junction 34)
  (junction 34) -> Wait3 [order 2]
  Wait3 -> (junction 34)
  (junction 34) -> DAC_D [order 1] : [count_5742 > 20]
  data: count_5742 data_store_memory; FLAG_5742 data_store_memory
  events: DAC_A_OUT output FUNCTION_CALL_EVENT; DAC_B_OUT output FUNCTION_CALL_EVENT; DAC_C_OUT output FUNCTION_CALL_EVENT; DAC_D_OUT output FUNCTION_CALL_EVENT

== matlab function TEST_IPM_2_0/INT/MAX5742/MAX1 ==
  data: Group input
  events: DACA_1 output FUNCTION_CALL_EVENT; DACB_1 output FUNCTION_CALL_EVENT; DACC_1 output FUNCTION_CALL_EVENT; DACD_1 output FUNCTION_CALL_EVENT; DACA_2 output FUNCTION_CALL_EVENT; DACB_2 output FUNCTION_CALL_EVENT; DACC_2 output FUNCTION_CALL_EVENT; DACD_2 output FUNCTION_CALL_EVENT
function MAX5742(Group)
persistent count
if isempty(count)
	count = uint16(1);
end
count = count + uint16(1);
if(Group == uint16(1))
    if(count == 1)
        DACA_1;
    elseif(count == 2)
        DACB_1;
    elseif(count == 3)
        DACC_1;
    else
        count = uint16(0);
        DACD_1;
    end
else
    if(count == 1)
        DACA_2;
    elseif(count == 2)
        DACB_2;
    elseif(count == 3)
        DACC_2;
    else
        count = uint16(0);
        DACD_2;
    end
end

== matlab function TEST_IPM_2_0/INT/Motor Control/Current_PI/MATLAB Function3 ==
  data: Umd input; udh output; Umq input; FRQ input; uqh output
function [udh,uqh] = HFI(Umd,Umq,FRQ)
persistent HFI_COUNT
if isempty(HFI_COUNT)
    HFI_COUNT = single(0);
end
HFI_COUNT = HFI_COUNT + single(2)*single(pi)*single(1e-4)*FRQ;
if(HFI_COUNT >= single(2)*single(pi))
    HFI_COUNT = HFI_COUNT - single(2)*single(pi);
end

udh = Umd * sin (HFI_COUNT);
uqh = Umq * cos (HFI_COUNT);

== matlab function TEST_IPM_2_0/INT/Motor Control/Current_PI/MATLAB Function5 ==
  data: Imd input; idh output; Imq input; FRQ input; iqh output
function [idh,iqh] = HFI(Imd,Imq,FRQ)
persistent HFI_COUNT
if isempty(HFI_COUNT)
    HFI_COUNT = single(0);
end
HFI_COUNT = HFI_COUNT + single(2)*single(pi)*single(1e-4)*FRQ;
if(HFI_COUNT >= single(2)*single(pi))
    HFI_COUNT = HFI_COUNT - single(2)*single(pi);
end

idh = Imd * sin (HFI_COUNT);
iqh = Imq * cos (HFI_COUNT);

== matlab function TEST_IPM_2_0/INT/GPIO UP/MATLAB Function2 ==
  data: IGBT_FAULT input; STOP data_store_memory; PROTECT data_store_memory
function DRIVE_FAULT(IGBT_FAULT)
global STOP PROTECT
if (IGBT_FAULT ~= uint16(63))
    STOP = uint16(1);
     PROTECT = uint16(bitor(PROTECT,uint16(16)));
end

== matlab function TEST_IPM_2_0/INT/Motor Control/TorqueMode/MATLAB Function2 ==
  data: Target input; Set_Point output; Step input; STOP data_store_memory
function Set_Point = RAMP_Control(Target,Step)
global STOP;

persistent Set_Point_Value;
if isempty(Set_Point_Value)
   Set_Point_Value = single(0);
end
if(Target >= Set_Point_Value)
	Set_Point_Value = Set_Point_Value + Step;
else
	Set_Point_Value = Set_Point_Value - Step;
end


if(abs(Target - Set_Point_Value) <= Step*2)
    Set_Point_Value = Target;
end


if(Set_Point_Value >= single(400))
    Set_Point_Value = single(400);
elseif(Set_Point_Value <= single(-400))
    Set_Point_Value = single(-400);
end
if(STOP ~= uint16(0))
    Set_Point_Value = single(0);
end
Set_Point = Set_Point_Value;
end

== matlab function TEST_IPM_2_0/INT/Read Rotor Position/SpeedCal/MATLAB Function1 ==
  data: theta input; speed output single; theta_old input; Ts_1kHz parameter
function speed = Est_Speed(theta,theta_old, Ts_1kHz)

error = (theta - theta_old);
if(error > pi)
    error = error - single(2)*single(pi);
elseif(error <- pi)
	error = error + single(2)*single(pi);
end
speed = error/(Ts_1kHz)*single(9.54929674)*single(0.25);
end

== matlab function TEST_IPM_2_0/INT/Motor Control/TorqueMode/MATLAB Function1 ==
  data: n input
  events: PI_Clear output FUNCTION_CALL_EVENT
function n_Protect(n)

    if(n < -300 || n > 300)
        PI_Clear;
    end
end

== matlab function TEST_IPM_2_0/INT/Motor Control/Current_PI/MATLAB Function6 ==
  data: IRef input; IFbk input; PROTECT data_store_memory; STOP data_store_memory
function DQCurrentProtect(IRef,IFbk)
global PROTECT STOP
if(abs(IRef - IFbk) >= 5)
    STOP = uint16(1);
    PROTECT = uint16(bitor(PROTECT,16)); 
end    
if(PROTECT ~= uint16(0))
    STOP = uint16(1);
end

== matlab function TEST_IPM_2_0/INT/Motor Control/Current_PI/MATLAB Function7 ==
  data: IRef input; IFbk input; PROTECT data_store_memory; STOP data_store_memory
function DQCurrentProtect(IRef,IFbk)
global PROTECT STOP
if(abs(IRef - IFbk) >= 5)
    STOP = uint16(1);
    PROTECT = uint16(bitor(PROTECT,16)); 
end    
if(PROTECT ~= uint16(0))
    STOP = uint16(1);
end
